simulink model "hinf_control_no_derivative_feedback_closed_loop_system"  (R2020b)
settings: Solver=VariableStepAuto  StartTime=0.0  StopTime=200  RelTol=1e-3
values from neighbouring files (symbols this model uses):
  COMMANDED_TORQUE_SATURATION = 0.05    [Workshop_MATLAB.m]
  COUPLING_COEFFICIENT = 0.5736    [Workshop_MATLAB.m]
  DISTURBANCE_TORQUE = 0.001    [Workshop_MATLAB.m]
  DISTURBANCE_TORQUE_DELAY = 100    [Workshop_MATLAB.m]
  FLEXIBLE_MODE_DAMPING_RATIO = 0.00495    [Workshop_MATLAB.m]
  FLEXIBLE_MODE_FREQUENCY = 2.6268    [Workshop_MATLAB.m]
  INITIAL_CONDITION_ON_STATE = 0.0001    [Workshop_MATLAB.m]
  MAXIMUM_TOLERABLE_POINTING_ERROR = 3.5*2*pi/360    (= 0.0610865238198)    [Workshop_MATLAB.m]
  MEASUREMENT_NOISE_VARIANCE = 10^(-9)    (= 1e-09)    [Workshop_MATLAB.m]
  REACTION_WHEEL_DYNAMICS_DENOMINATOR = [1 2.400 0.763]    [Workshop_MATLAB.m]
  REACTION_WHEEL_DYNAMICS_NUMERATOR = REACTION_WHEEL_INERTIA*[1.214 0.763 0]    [Workshop_MATLAB.m]
  REACTION_WHEEL_INERTIA = 0.0004    [Workshop_MATLAB.m]
  REACTION_WHEEL_VELOCITY_SATURATION = 2800*2*pi/60    (= 293.215314335)    [Workshop_MATLAB.m]
  SATELLITE_INERTIA = 31.38    [Workshop_MATLAB.m]
  STAR_TRACKER_NOISE_DELAY = 160    [Workshop_MATLAB.m]
undefined symbols (not defined in the file or in its folder): hinfControlNoDerivativeFeedbackStateSpace, TARGET_SECOND_ORDER
settings Model: Creator=WLCG  LastModifiedBy=WLCG

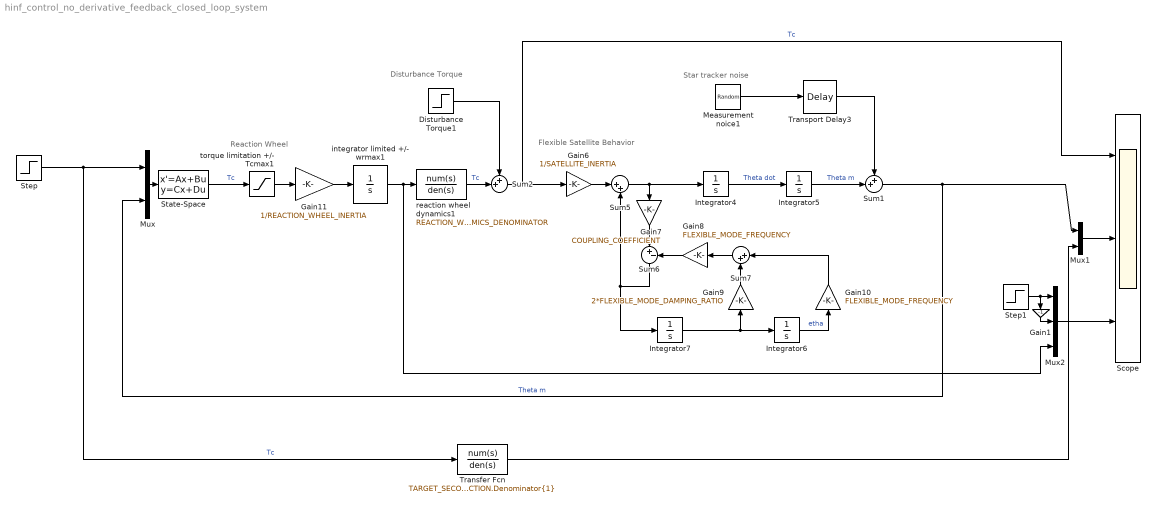
== system hinf_control_no_derivative_feedback_closed_loop_system ==
  note: Disturbance Torque
  note: Star tracker noise
  note: Flexible Satellite Behavior
  note: Reaction Wheel
  Disturbance Torque1 : Step  Time=DISTURBANCE_TORQUE_DELAY  After=DISTURBANCE_TORQUE  SampleTime=0
  Gain1 : Gain  Gain=-1
  Gain10 : Gain  Gain=FLEXIBLE_MODE_FREQUENCY
  Gain11 : Gain  Gain=1/REACTION_WHEEL_INERTIA
  Gain6 : Gain  Gain=1/SATELLITE_INERTIA
  Gain7 : Gain  Gain=COUPLING_COEFFICIENT
  Gain8 : Gain  Gain=FLEXIBLE_MODE_FREQUENCY
  Gain9 : Gain  Gain=2*FLEXIBLE_MODE_DAMPING_RATIO
  Integrator4 : Integrator
  Integrator5 : Integrator
  Integrator6 : Integrator  InitialCondition=INITIAL_CONDITION_ON_STATE
  Integrator7 : Integrator
  Measurement noice1 : RandomNumber  Variance=MEASUREMENT_NOISE_VARIANCE  SampleTime=0.01
  Mux : Mux  Inputs=2
  Mux1 : Mux  Inputs=2
  Mux2 : Mux  Inputs=3
  Scope : Scope  NumInputPorts=3
  State-Space : StateSpace  A=hinfControlNoDerivativeFeedbackStateSpace.A  B=hinfControlNoDerivativeFeedbackStateSpace.B  C=hinfControlNoDerivativeFeedbackStateSpace.C  D=hinfControlNoDerivativeFeedbackStateSpace.D  InitialCondition=0
  Step : Step  Time=0  After=MAXIMUM_TOLERABLE_POINTING_ERROR  SampleTime=0
  Step1 : Step  Time=0  After=REACTION_WHEEL_VELOCITY_SATURATION  SampleTime=0
  Sum1 : Sum  Inputs=++|
  Sum2 : Sum  Inputs=++|
  Sum5 : Sum  Inputs=|++
  Sum6 : Sum  Inputs=|+-
  Sum7 : Sum  Inputs=|++
  Transfer Fcn : TransferFcn  Numerator=TARGET_SECOND_ORDER.TRANSFER_FUNCTION.Numerator{1}  Denominator=TARGET_SECOND_ORDER.TRANSFER_FUNCTION.Denominator{1}
  Transport Delay3 : TransportDelay  DelayTime=STAR_TRACKER_NOISE_DELAY
  integrator limited +/- wrmax1 : Integrator  LimitOutput=on  UpperSaturationLimit=REACTION_WHEEL_VELOCITY_SATURATION  LowerSaturationLimit=-REACTION_WHEEL_VELOCITY_SATURATION
  reaction wheel dynamics1 : TransferFcn  Numerator=REACTION_WHEEL_DYNAMICS_NUMERATOR  Denominator=REACTION_WHEEL_DYNAMICS_DENOMINATOR
  torque limitation +/- Tcmax1 : Saturate  UpperLimit=COMMANDED_TORQUE_SATURATION  LowerLimit=-COMMANDED_TORQUE_SATURATION
  wires:
  Gain7/1 -> Sum6/1
  Gain9/1 -> Sum7/2
  Sum7/1 -> Gain8/1
  Sum1/1 -> Mux/2, Mux1/1  "Theta m"
  Gain10/1 -> Sum7/1
  Sum2/1 -> Scope/1, Gain6/1  "Tc"
  Gain8/1 -> Sum6/2
  Integrator4/1 -> Integrator5/1  "Theta dot"
  Gain6/1 -> Sum5/1
  Gain11/1 -> integrator limited +/- wrmax1/1
  Sum5/1 -> Integrator4/1, Gain7/1
  Integrator6/1 -> Gain10/1  "etha"
  Integrator7/1 -> Integrator6/1, Gain9/1
  integrator limited +/- wrmax1/1 -> Mux2/3, reaction wheel dynamics1/1
  Sum6/1 -> Integrator7/1, Sum5/2
  State-Space/1 -> torque limitation +/- Tcmax1/1  "Tc"
  Step/1 -> Transfer Fcn/1, Mux/1  "Tc"
  Transfer Fcn/1 -> Mux1/2
  Mux/1 -> State-Space/1
  torque limitation +/- Tcmax1/1 -> Gain11/1
  Measurement noice1/1 -> Transport Delay3/1
  Integrator5/1 -> Sum1/2  "Theta m"
  Transport Delay3/1 -> Sum1/1
  Disturbance Torque1/1 -> Sum2/1
  reaction wheel dynamics1/1 -> Sum2/2  "Tc"
  Mux1/1 -> Scope/2
  Step1/1 -> Gain1/1, Mux2/1
  Gain1/1 -> Mux2/2
  Mux2/1 -> Scope/3
